simulink model "project_1_part4"  (R2021b)
settings: Solver=ode3  StartTime=0.0  StopTime=10.0  FixedStep=0.01  RelTol=1e-3
settings Model: Creator=jlkbo  LastModifiedBy=jlkbo

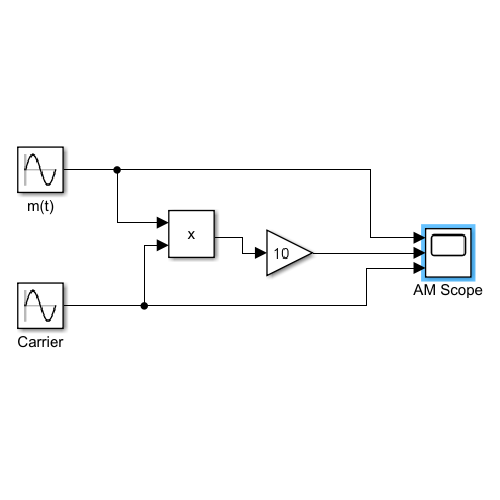
[thumbnail: Simulink's stored preview of the top-level diagram]
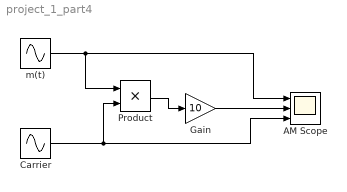
== system project_1_part4 ==
  AM Scope : Scope  NumInputPorts=3
  Carrier : Sin  Amplitude=20  Frequency=5  SampleTime=0
  Gain : Gain  Gain=10
  Product : Product
  m(t) : Sin  Amplitude=2  Frequency=2*3.1416  SampleTime=0
  wires:
  m(t)/1 -> AM Scope/1, Product/1
  Carrier/1 -> AM Scope/3, Product/2
  Product/1 -> Gain/1
  Gain/1 -> AM Scope/2
